simulink model "gridconnectedpvarray"  (R2023b)
settings: Solver=FixedStepDiscrete  StartTime=0.0  StopTime=2.5  RelTol=1e-3
PreLoadFcn:
  | Ts_Power=1e-6;
  | Ts_Control=100e-6;
InitFcn:
  | Ts_Power=1e-6;
  | Ts_Control=100e-6;
undefined symbols (not defined in the file): D1, Delta, DiscIntNeverNeededParam
libraries: spsSeriesRLCBranchLib x5, spsMeanLib x3, spsThreePhaseTransformerTwoWindingsLib x2, spsDistributedParametersLineLib x2, spsThreePhaseParallelRLCLoadLib x2, spsFourierLib x2, slpidlib x2, spsabctodq0Lib x2, spsVoltageMeasurementLib x2, spsThreePhaseSeriesRLCLoadLib x1, spsThreeLevelBridgeLib x1, spsThreePhaseSourceLib x1
(part 2 of 2)

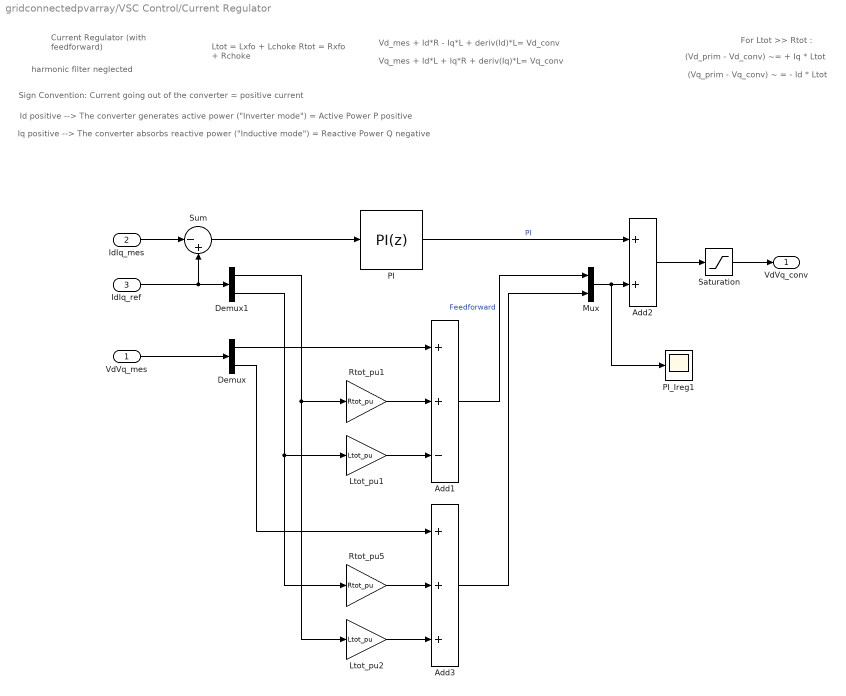
== system gridconnectedpvarray/VSC Control/Current Regulator ==
  note: harmonic filter neglected
  note: Vd_mes + Id*R - Iq*L + deriv(Id)*L= Vd_conv
  note: Vq_mes + Id*L + Iq*R + deriv(Iq)*L= Vq_conv
  note: Current Regulator
      | (with feedforward)
  note: Sign Convention: Current going out of the converter = positive current
  note: Iq positive --> The converter absorbs reactive power ("Inductive mode") = Reactive Power Q negative
  note: Id positive --> The converter generates active power ("Inverter mode") = Active Power P positive
  note: Ltot = Lxfo + Lchoke
      | Rtot = Rxfo + Rchoke
  note: (Vd_prim - Vd_conv) ~= + Iq * Ltot
  note: (Vq_prim - Vq_conv) ~ = - Id * Ltot
  note: For Ltot >> Rtot :
  VdVq_mes : Inport  PortDimensions=2
  IdIq_mes : Inport  Port=2  PortDimensions=2
  IdIq_ref : Inport  Port=3  PortDimensions=2
  Add1 : Sum  Inputs=++-
  Add2 : Sum
  Add3 : Sum  Inputs=+++
  Demux : Demux  Outputs=2
  Demux1 : Demux  Outputs=2
  Ltot_pu1 : Gain  Gain=Ltot_pu  SaturateOnIntegerOverflow=on  OutDataTypeStr=Inherit: Same as input  ParamDataTypeStr=Inherit: Same as input
  Ltot_pu2 : Gain  Gain=Ltot_pu  SaturateOnIntegerOverflow=on  OutDataTypeStr=Inherit: Same as input  ParamDataTypeStr=Inherit: Same as input
  Mux : Mux  Inputs=2
  PI : slpidlib/PID Controller  Controller=PI  Form=Parallel  TimeDomain=Discrete-time  UseExternalTs=off  SampleTime=Ts  IntegratorMethod=Forward Euler  FilterMethod=Forward Euler  ControllerParametersSource=internal  P=Kp_Ireg  I=Ki_Ireg  UseKiTs=off  D=0  N=100  UseFilter=on  TunerSelectOption=Transfer Function Based (PID Tuner App)  InitialConditionSource=internal  InitialConditionForIntegrator=0  InitialConditionForFilter=0  DifferentiatorICPrevScaledInput=0  ExternalReset=none  TrackingMode=off  Kt=1  LimitOutput=on  SatLimitsSource=internal  UpperSaturationLimit=2  LowerSaturationLimit=-2  LinearizeAsGain=off  AntiWindupMode=none  Kb=1  LimitIntegrator=off  UpperIntegratorSaturationLimit=inf  LowerIntegratorSaturationLimit=-inf  POutMin=[]  POutMax=[]  IOutMin=[]  IOutMax=[]  DOutMin=[]  DOutMax=[]  NOutMin=[]  NOutMax=[]  SumOutMin=[]  SumOutMax=[]  SaturationOutMin=[]  SaturationOutMax=[]  PParamMin=[]  PParamMax=[]  IParamMin=[]  IParamMax=[]  DParamMin=[]  DParamMax=[]  NParamMin=[]  NParamMax=[]  KbParamMin=[]  KbParamMax=[]  KtParamMin=[]  KtParamMax=[]  KbOutMin=[]  KbOutMax=[]  KtOutMin=[]  KtOutMax=[]  IntegratorOutMin=[]  IntegratorOutMax=[]  FilterOutMin=[]  FilterOutMax=[]  SumI1OutMin=[]  SumI1OutMax=[]  SumI2OutMin=[]  SumI2OutMax=[]  SumI3OutMin=[]  SumI3OutMax=[]  SumI4OutMin=[]  SumI4OutMax=[]  SumDOutMin=[]  SumDOutMax=[]  DifferentiatorOutMin=[]  DifferentiatorOutMax=[]  FilterDiffOutCoefMin=[]  FilterDiffOutCoefMax=[]  ReciprocalOutMin=[]  ReciprocalOutMax=[]  SumDenOutMin=[]  SumDenOutMax=[]  SumNumOutMin=[]  SumNumOutMax=[]  DivideOutMin=[]  DivideOutMax=[]  UdiffTsProdOutMin=[]  UdiffTsProdOutMax=[]  NTsProdOutMin=[]  NTsProdOutMax=[]  UintegralTsProdOutMin=[]  UintegralTsProdOutMax=[]  UngainTsProdOutMin=[]  UngainTsProdOutMax=[]  ClampingZeroOutDataTypeStr=Inherit: Inherit via back propagation  ClampingZeroOutMin=[]  ClampingZeroOutMax=[]  FilterDenConstantOutDataTypeStr=Inherit: Inherit via back propagation  FilterDenConstantOutMin=[]  FilterDenConstantOutMax=[]  PCopyOutDataTypeStr=Inherit: Inherit via back propagation  PCopyOutMin=[]  PCopyOutMax=[]  NCopyOutDataTypeStr=Inherit: Inherit via back propagation  NCopyOutMin=[]  NCopyOutMax=[]  IntegratorContinuousStateAttributes=''  IntegratorStateMustResolveToSignalObject=off  IntegratorRTWStateStorageClass=Auto  FilterContinuousStateAttributes=''  FilterStateMustResolveToSignalObject=off  FilterRTWStateStorageClass=Auto  ParallelPVariant=InternalParameters  IdealPVariant=Disabled  IVariant=InternalParameters  DVariant=Disabled  IntegratorVariant=Discrete  SatVariant=Enabled  AWVariant=Passthrough  PCopyVariant=Disabled  TRVariant=Disabled  FdbkBlocksVariant=Forward  IdealPFdbkVariant=Disabled  SatFdbkVariant=Disabled  DerivativeFilterVariant=Disabled  NVariant=Disabled  NCopyVariant=Disabled_SignalSpec  FilterICVariant=Disabled  IntegratorICVariant=InternalICs  ExternalResetVariant=Disabled  TRSumVariant=Passthrough  SumFdbkVariant=Disabled  SumVariant=Sum_PI  TsampFilterVariant=InternalTs  TsampNgainVariant=Passthrough  TsampIntegralVariant=Disabled_SignalSpec  ExternalSaturationOutDataTypeStr=Inherit: Same as second input
  PI_Ireg1 : Scope
  Rtot_pu1 : Gain  Gain=Rtot_pu  SaturateOnIntegerOverflow=on  OutDataTypeStr=Inherit: Same as input  ParamDataTypeStr=Inherit: Same as input
  Rtot_pu5 : Gain  Gain=Rtot_pu  SaturateOnIntegerOverflow=on  OutDataTypeStr=Inherit: Same as input  ParamDataTypeStr=Inherit: Same as input
  Saturation : Saturate  UpperLimit=2  LowerLimit=-2
  Sum : Sum  Inputs=|-+
  VdVq_conv : Outport  VectorParamsAs1DForOutWhenUnconnected=off
  wires:
  Mux/1 -> PI_Ireg1/1, Add2/2
  PI/1 -> Add2/1  "PI"
  Sum/1 -> PI/1
  IdIq_ref/1 -> Sum/2, Demux1/1
  IdIq_mes/1 -> Sum/1
  Add2/1 -> Saturation/1
  Saturation/1 -> VdVq_conv/1
  VdVq_mes/1 -> Demux/1
  Demux/1 -> Add1/1
  Rtot_pu1/1 -> Add1/2
  Demux1/1 -> Rtot_pu1/1, Ltot_pu2/1
  Ltot_pu1/1 -> Add1/3
  Demux1/2 -> Ltot_pu1/1, Rtot_pu5/1
  Rtot_pu5/1 -> Add3/2
  Ltot_pu2/1 -> Add3/3
  Add1/1 -> Mux/1  "Feedforward"
  Demux/2 -> Add3/1
  Add3/1 -> Mux/2

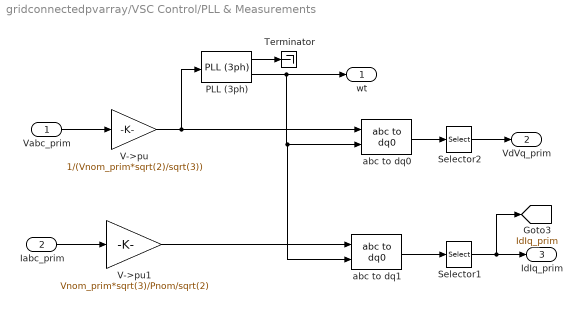
== system gridconnectedpvarray/VSC Control/PLL & Measurements ==
  Vabc_prim : Inport
  Iabc_prim : Inport  Port=2
  PLL (3ph) : spsPLL3phLib/PLL (3ph)  Fmin=45  Par_Init="[-0.57  Fnom]"  ParK=[180, 3200, 1]  TcD=1e-4  MaxRateChangeFreq=12  FilterCutOffFreq=25  Ts=Ts  AGC=on
  Selector1 : Selector  InputPortWidth=3  IndexOptions=Index vector (dialog)  Indices=[1 2]  OutputSizes=1
  Selector2 : Selector  InputPortWidth=3  IndexOptions=Index vector (dialog)  Indices=[1 2]  OutputSizes=1
  Terminator : Terminator
  V->pu : Gain  Gain=1/(Vnom_prim*sqrt(2)/sqrt(3))  SaturateOnIntegerOverflow=on  OutDataTypeStr=Inherit: Same as input  ParamDataTypeStr=Inherit: Same as input
  V->pu1 : Gain  Gain=Vnom_prim*sqrt(3)/Pnom/sqrt(2)  SaturateOnIntegerOverflow=on  OutDataTypeStr=Inherit: Same as input  ParamDataTypeStr=Inherit: Same as input
  abc to dq0 : spsabctodq0Lib/abc to dq0  Alignment=90 degrees behind phase A axis
  abc to dq1 : spsabctodq0Lib/abc to dq0  Alignment=90 degrees behind phase A axis
  wt : Outport  VectorParamsAs1DForOutWhenUnconnected=off
  VdVq_prim : Outport  Port=2  VectorParamsAs1DForOutWhenUnconnected=off
  IdIq_prim : Outport  Port=3  VectorParamsAs1DForOutWhenUnconnected=off
  tag scope: IdIq_prim=global
  wires:
  V->pu1/1 -> abc to dq1/1
  V->pu/1 -> PLL (3ph)/1, abc to dq0/1
  abc to dq1/1 -> Selector1/1
  Vabc_prim/1 -> V->pu/1
  Iabc_prim/1 -> V->pu1/1
  abc to dq0/1 -> Selector2/1
  Selector2/1 -> VdVq_prim/1
  Selector1/1 -> [IdIq_prim], IdIq_prim/1
  PLL (3ph)/2 -> wt/1, abc to dq1/2, abc to dq0/2
  PLL (3ph)/1 -> Terminator/1

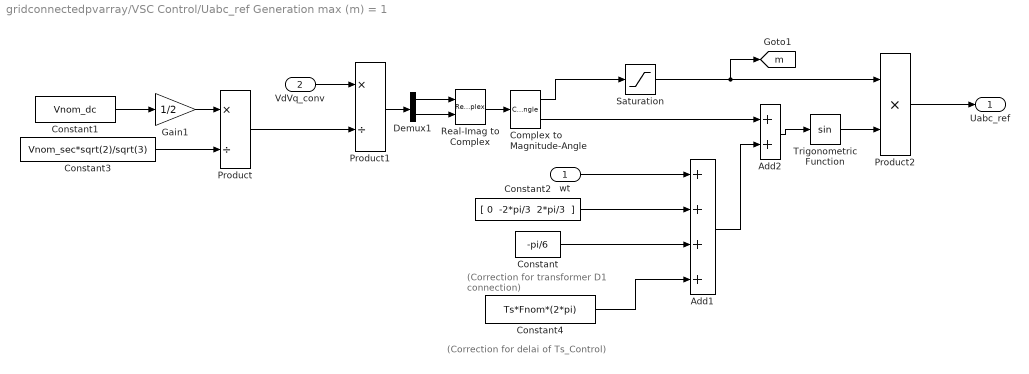
== system gridconnectedpvarray/VSC Control/Uabc_ref Generation max (m) = 1 ==
  note: (Correction for transformer
      |  D1 connection)
  note: (Correction for delai of Ts_Control)
  wt : Inport
  VdVq_conv : Inport  Port=2
  Add1 : Sum  Inputs=++++
  Add2 : Sum
  Complex to Magnitude-Angle : ComplexToMagnitudeAngle
  Constant : Constant  Value=-pi/6
  Constant1 : Constant  Value=Vnom_dc
  Constant2 : Constant  Value="[ 0  -2*pi/3  2*pi/3  ]"
  Constant3 : Constant  Value=Vnom_sec*sqrt(2)/sqrt(3)
  Constant4 : Constant  Value=Ts*Fnom*(2*pi)
  Demux1 : Demux  Outputs=2
  Gain1 : Gain  Gain=1/2
  Product : Product  Inputs=*/  RndMeth=Zero
  Product1 : Product  Inputs=*/  RndMeth=Zero
  Product2 : Product  Inputs=**  RndMeth=Zero
  Real-Imag to Complex : RealImagToComplex
  Saturation : Saturate  UpperLimit=1  LowerLimit=0
  Trigonometric Function : Trigonometry
  Uabc_ref : Outport  VectorParamsAs1DForOutWhenUnconnected=off
  tag scope: m=global
  wires:
  Complex to Magnitude-Angle/1 -> Saturation/1
  Constant1/1 -> Gain1/1
  VdVq_conv/1 -> Product1/1
  Product1/1 -> Demux1/1
  Gain1/1 -> Product/1
  Real-Imag to Complex/1 -> Complex to Magnitude-Angle/1
  Demux1/1 -> Real-Imag to Complex/1
  Demux1/2 -> Real-Imag to Complex/2
  Constant2/1 -> Add1/2
  Constant/1 -> Add1/3
  Constant3/1 -> Product/2
  Product/1 -> Product1/2
  Complex to Magnitude-Angle/2 -> Add2/1
  Add1/1 -> Add2/2
  Add2/1 -> Trigonometric Function/1
  Saturation/1 -> [m], Product2/1
  Trigonometric Function/1 -> Product2/2
  Product2/1 -> Uabc_ref/1
  wt/1 -> Add1/1
  Constant4/1 -> Add1/4

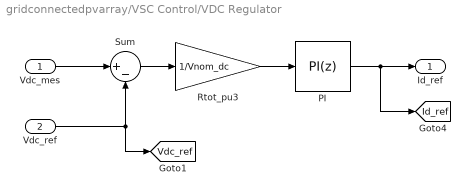
== system gridconnectedpvarray/VSC Control/VDC Regulator ==
  Vdc_mes : Inport  PortDimensions=1
  Vdc_ref : Inport  Port=2  PortDimensions=1
  PI : slpidlib/PID Controller  Controller=PI  Form=Parallel  TimeDomain=Discrete-time  UseExternalTs=off  SampleTime=Ts  IntegratorMethod=Trapezoidal  FilterMethod=Forward Euler  ControllerParametersSource=internal  P=Kp_VDCreg  I=Ki_VDCreg  UseKiTs=off  D=0  N=100  UseFilter=on  TunerSelectOption=Transfer Function Based (PID Tuner App)  InitialConditionSource=internal  InitialConditionForIntegrator=0  InitialConditionForFilter=0  DifferentiatorICPrevScaledInput=0  ExternalReset=none  TrackingMode=off  Kt=1  LimitOutput=on  SatLimitsSource=internal  UpperSaturationLimit=1.5  LowerSaturationLimit=-1.5  LinearizeAsGain=off  AntiWindupMode=none  Kb=1  LimitIntegrator=off  UpperIntegratorSaturationLimit=inf  LowerIntegratorSaturationLimit=-inf  POutMin=[]  POutMax=[]  IOutMin=[]  IOutMax=[]  DOutMin=[]  DOutMax=[]  NOutMin=[]  NOutMax=[]  SumOutMin=[]  SumOutMax=[]  SaturationOutMin=[]  SaturationOutMax=[]  PParamMin=[]  PParamMax=[]  IParamMin=[]  IParamMax=[]  DParamMin=[]  DParamMax=[]  NParamMin=[]  NParamMax=[]  KbParamMin=[]  KbParamMax=[]  KtParamMin=[]  KtParamMax=[]  KbOutMin=[]  KbOutMax=[]  KtOutMin=[]  KtOutMax=[]  IntegratorOutMin=[]  IntegratorOutMax=[]  FilterOutMin=[]  FilterOutMax=[]  SumI1OutMin=[]  SumI1OutMax=[]  SumI2OutMin=[]  SumI2OutMax=[]  SumI3OutMin=[]  SumI3OutMax=[]  SumI4OutMin=[]  SumI4OutMax=[]  SumDOutMin=[]  SumDOutMax=[]  DifferentiatorOutMin=[]  DifferentiatorOutMax=[]  FilterDiffOutCoefMin=[]  FilterDiffOutCoefMax=[]  ReciprocalOutMin=[]  ReciprocalOutMax=[]  SumDenOutMin=[]  SumDenOutMax=[]  SumNumOutMin=[]  SumNumOutMax=[]  DivideOutMin=[]  DivideOutMax=[]  UdiffTsProdOutMin=[]  UdiffTsProdOutMax=[]  NTsProdOutMin=[]  NTsProdOutMax=[]  UintegralTsProdOutMin=[]  UintegralTsProdOutMax=[]  UngainTsProdOutMin=[]  UngainTsProdOutMax=[]  ClampingZeroOutDataTypeStr=Inherit: Inherit via back propagation  ClampingZeroOutMin=[]  ClampingZeroOutMax=[]  FilterDenConstantOutDataTypeStr=Inherit: Inherit via back propagation  FilterDenConstantOutMin=[]  FilterDenConstantOutMax=[]  PCopyOutDataTypeStr=Inherit: Inherit via back propagation  PCopyOutMin=[]  PCopyOutMax=[]  NCopyOutDataTypeStr=Inherit: Inherit via back propagation  NCopyOutMin=[]  NCopyOutMax=[]  IntegratorContinuousStateAttributes=''  IntegratorStateMustResolveToSignalObject=off  IntegratorRTWStateStorageClass=Auto  FilterContinuousStateAttributes=''  FilterStateMustResolveToSignalObject=off  FilterRTWStateStorageClass=Auto  ParallelPVariant=InternalParameters  IdealPVariant=Disabled  IVariant=InternalParameters  DVariant=Disabled  IntegratorVariant=Discrete  SatVariant=Enabled  AWVariant=Passthrough  PCopyVariant=Disabled  TRVariant=Disabled  FdbkBlocksVariant=Forward  IdealPFdbkVariant=Disabled  SatFdbkVariant=Disabled  DerivativeFilterVariant=Disabled  NVariant=Disabled  NCopyVariant=Disabled_SignalSpec  FilterICVariant=Disabled  IntegratorICVariant=InternalICs  ExternalResetVariant=Disabled  TRSumVariant=Passthrough  SumFdbkVariant=Disabled  SumVariant=Sum_PI  TsampFilterVariant=InternalTs  TsampNgainVariant=Passthrough  TsampIntegralVariant=Disabled_SignalSpec  ExternalSaturationOutDataTypeStr=Inherit: Same as second input
  Rtot_pu3 : Gain  Gain=1/Vnom_dc  SaturateOnIntegerOverflow=on  OutDataTypeStr=Inherit: Same as input  ParamDataTypeStr=Inherit: Same as input
  Sum : Sum  Inputs=|+-
  Id_ref : Outport  SampleTime=Ts  InitialOutput=0  VectorParamsAs1DForOutWhenUnconnected=off
  tag scope: Id_ref=global, Vdc_ref=global
  wires:
  Sum/1 -> Rtot_pu3/1
  Vdc_mes/1 -> Sum/1
  Vdc_ref/1 -> Sum/2, [Vdc_ref]
  Rtot_pu3/1 -> PI/1
  PI/1 -> [Id_ref], Id_ref/1
